simulink model "ball_beam_openloop"  (R2024a)
settings: Solver=VariableStepAuto  StartTime=0.0  StopTime=10.0  RelTol=1e-3
settings Model: Creator=jorda  LastModifiedBy=jorda

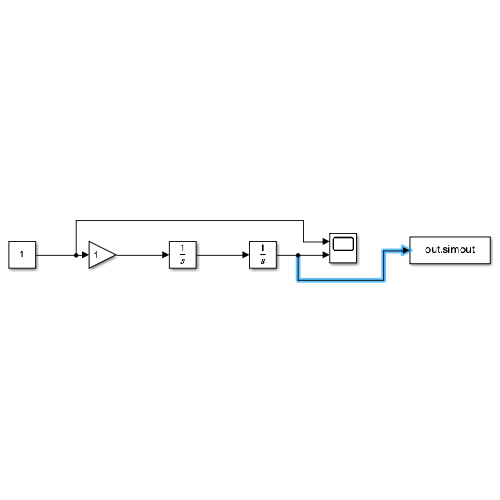
[thumbnail: Simulink's stored preview of the top-level diagram]
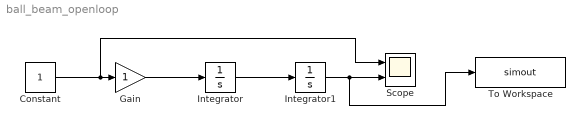
== system ball_beam_openloop ==
  Constant : Constant
  Gain : Gain
  Integrator : Integrator
  Integrator1 : Integrator
  Scope : Scope  NumInputPorts=2
  To Workspace : ToWorkspace  VariableName=simout  SaveFormat=Timeseries  SampleTime=-1
  wires:
  Constant/1 -> Scope/1, Gain/1
  Gain/1 -> Integrator/1
  Integrator/1 -> Integrator1/1
  Integrator1/1 -> To Workspace/1, Scope/2
